simulink model "USBlvbo"  (R2017b)
settings: Solver=VariableStepAuto  StartTime=0.0  StopTime=10.0  RelTol=1e-3
undefined symbols (not defined in the file or in its folder): xy1, zb1
libraries: dsparch4 x3
settings Model: Creator=DELL  LastModifiedBy=DELL

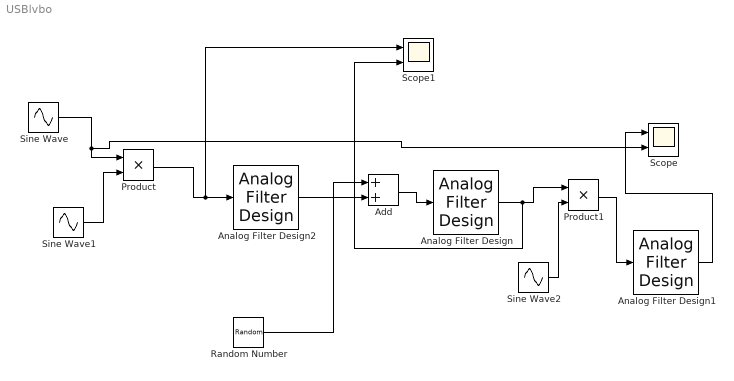
== system USBlvbo ==
  Add : Sum
  Analog Filter Design : dsparch4/Analog Filter Design  method=Butterworth  filttype=Bandpass  N=8  Wlo=100  Whi=110  Rp=2  Rs=40
  Analog Filter Design1 : dsparch4/Analog Filter Design  method=Butterworth  filttype=Lowpass  N=8  Wlo=10  Whi=80  Rp=2  Rs=40
  Analog Filter Design2 : dsparch4/Analog Filter Design  method=Butterworth  filttype=Bandpass  N=8  Wlo=100  Whi=110  Rp=2  Rs=40
  Product : Product
  Product1 : Product
  Random Number : RandomNumber  Variance=0.01  SampleTime=0.1
  Scope : Scope  NumInputPorts=2
  Scope1 : Scope  NumInputPorts=2
  Sine Wave : Sin  Frequency=xy1  SampleTime=0
  Sine Wave1 : Sin  Frequency=zb1  SampleTime=0
  Sine Wave2 : Sin  Frequency=zb1  SampleTime=0
  wires:
  Sine Wave1/1 -> Product/2
  Sine Wave/1 -> Scope/2, Product/1
  Analog Filter Design2/1 -> Add/2
  Product/1 -> Scope1/1, Analog Filter Design2/1
  Random Number/1 -> Add/1
  Add/1 -> Analog Filter Design/1
  Analog Filter Design/1 -> Scope1/2, Product1/1
  Sine Wave2/1 -> Product1/2
  Product1/1 -> Analog Filter Design1/1
  Analog Filter Design1/1 -> Scope/1
